simulink model "spike_generator"  (R2020b)
settings: Solver=FixedStepDiscrete  StartTime=0.0  StopTime=stopTime  RelTol=1e-3
InitFcn:
  | initCallback
StopFcn:
  | stopCallback
values from neighbouring files (symbols this model uses):
  nSites = 4    [Spike_Generator_Test_Parameters.m]
  tabs = 0.6e-3    (= 0.0006)    [Spike_Generator_Test_Parameters.m]
  trel = 0.6e-3    (= 0.0006)    [Spike_Generator_Test_Parameters.m]
undefined symbols (not defined in the file or in its folder): mp
settings Model: Creator=Ross  LastModifiedBy=tyler
settings DataIOCC: ReturnWorkspaceOutputs=off
settings OptimizationCC: BlockReduction=off  ConditionallyExecuteInputs=off  DefaultParameterBehavior=Inlined
settings DebuggingCC: ReadBeforeWriteMsg=DisableAll  WriteAfterWriteMsg=DisableAll  WriteAfterReadMsg=DisableAll  AlgebraicLoopMsg=error  MultiTaskDSMMsg=none  SingleTaskRateTransMsg=error  PregeneratedLibrarySubsystemCodeDiagnostic=none  ArithmeticOperatorsInVariantConditions=warning
settings HardwareCC: ProdBitPerPointer=32  ProdBitPerSizeT=32  ProdBitPerPtrDiffT=32  ProdLargestAtomicFloat=None  ProdIntDivRoundTo=Undefined  ProdEndianess=Unspecified  ProdWordSize=32  ProdHWDeviceType=ASIC/FPGA->ASIC/FPGA  TargetBitPerPointer=64  TargetBitPerSizeT=64  TargetBitPerPtrDiffT=64  TargetLongLongMode=on  TargetIntDivRoundTo=Zero  TargetEndianess=LittleEndian  TargetWordSize=64  TargetHWDeviceType=Custom Processor->MATLAB Host Computer  ProdEqTarget=off
settings ModelReferenceCC: UpdateModelReferenceTargets=IfOutOfDate
settings SFSimCC: SFSimEcho=off  SimUseLocalCustomCode=off  CustomCodeUndefinedFunction=UseInterfaceOnly
settings RTWCC: RTWUseLocalCustomCode=off

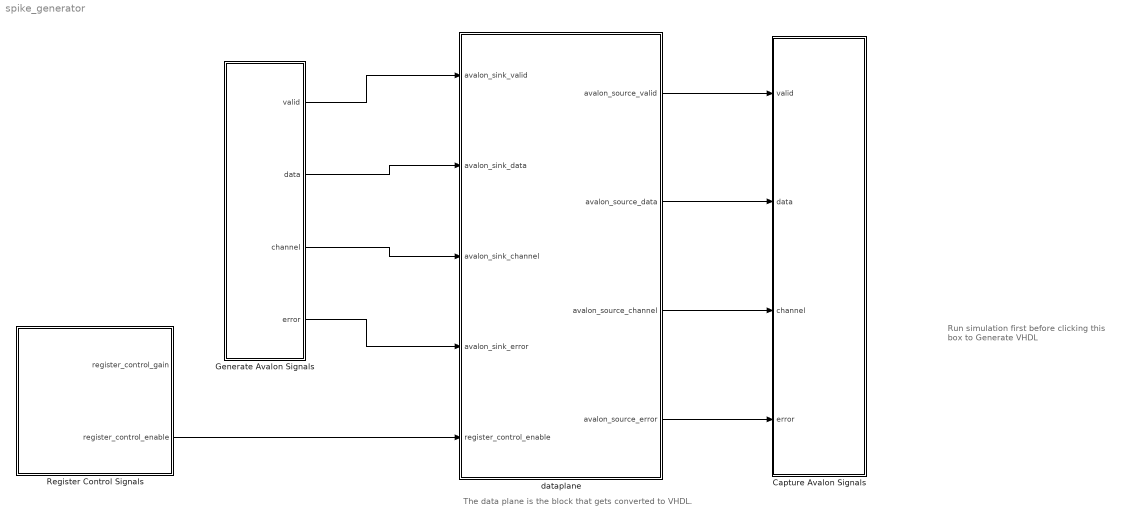
== system spike_generator ==
  note: The data plane is the block that gets converted to VHDL.
  note: Run simulation first
      | before clicking this box to
      | Generate VHDL
  Capture Avalon Signals : Subsystem
  Generate Avalon Signals : Subsystem
  Register Control Signals : Subsystem
  dataplane : Subsystem  TreatAsAtomicUnit=on
  wires:
  Generate Avalon Signals/2(data) -> dataplane/2(avalon_sink_data)
  Generate Avalon Signals/1(valid) -> dataplane/1(avalon_sink_valid)
  Generate Avalon Signals/3(channel) -> dataplane/3(avalon_sink_channel)
  Generate Avalon Signals/4(error) -> dataplane/4(avalon_sink_error)
  dataplane/2(avalon_source_data) -> Capture Avalon Signals/2(data)
  dataplane/1(avalon_source_valid) -> Capture Avalon Signals/1(valid)
  dataplane/3(avalon_source_channel) -> Capture Avalon Signals/3(channel)
  dataplane/4(avalon_source_error) -> Capture Avalon Signals/4(error)
  Register Control Signals/2(register_control_enable) -> dataplane/5(register_control_enable)

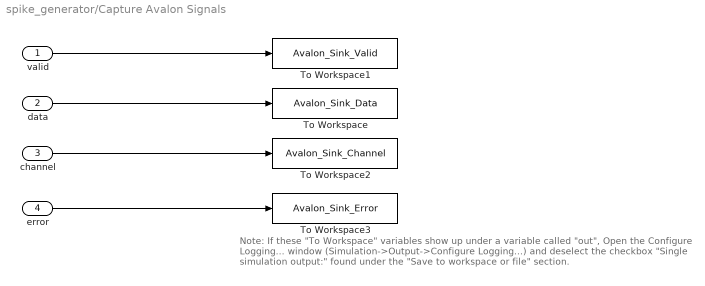
== system spike_generator/Capture Avalon Signals ==
  note: Note:  If these "To Workspace" variables show up under a variable called "out",
      | Open the Configure Logging... window (Simulation->Output->Configure Logging...)
      | and deselect the checkbox "Single simulation output:" found under the "Save to workspace or file" section.
  valid : Inport
  data : Inport  Port=2
  channel : Inport  Port=3
  error : Inport  Port=4
  To Workspace : ToWorkspace  VariableName=Avalon_Sink_Data  SaveFormat=Timeseries  SampleTime=-1
  To Workspace1 : ToWorkspace  VariableName=Avalon_Sink_Valid  SaveFormat=Timeseries  SampleTime=-1
  To Workspace2 : ToWorkspace  VariableName=Avalon_Sink_Channel  SaveFormat=Timeseries  SampleTime=-1
  To Workspace3 : ToWorkspace  VariableName=Avalon_Sink_Error  SaveFormat=Timeseries  SampleTime=-1
  wires:
  data/1 -> To Workspace/1
  valid/1 -> To Workspace1/1
  error/1 -> To Workspace3/1
  channel/1 -> To Workspace2/1

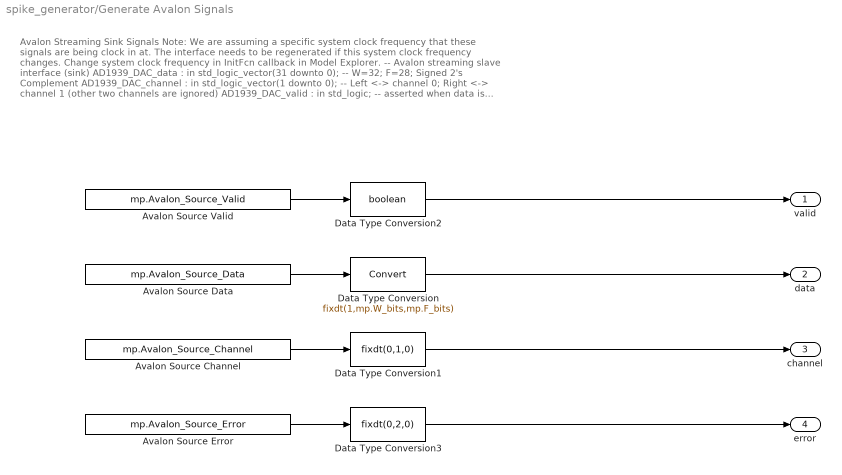
== system spike_generator/Generate Avalon Signals ==
  note: Avalon Streaming Sink Signals
      | Note: We are assuming a specific system clock frequency that these signals are being clock in at.
      | The interface needs to be regenerated if this system clock frequency changes. Change system clock frequency in InitFcn callback in Model Explorer.
      |
      | -- Avalon streaming slave interface (sink)
      | AD1939_DAC_data : in std_logic_vector(31 downto 0); -- W=32; F=28; Signed 2's Complement
      | AD1939_DAC_channel : in std_logic_vector(1 downto 0); -- Left <-> channel 0; Right <-> channel 1 (other two channels are ignored)
      | AD1939_DAC_valid : in std_logic; -- asserted when data is valid
      | AD1939_DAC_error : in std_logic_vector(1 downto 0) -- error channel is ignored, assumed to be error free at this point
      |
      | For more information on the data-channel-valid protocol, s ee chapter 5 in Intel's Avalon Interfaced Specification (p. 40) at https://www.intel.com/content/dam/www/programmable/us/en/pdfs/literature/manual/mnl_avalon_spec.pdf
  Avalon Source Channel : FromWorkspace  VariableName=mp.Avalon_Source_Channel  OutDataTypeStr=double  SampleTime=mp.Ts_sim
  "Avalon Source Data " : FromWorkspace  VariableName=mp.Avalon_Source_Data  OutDataTypeStr=double  SampleTime=mp.Ts_sim
  Avalon Source Error : FromWorkspace  VariableName=mp.Avalon_Source_Error  OutDataTypeStr=double  SampleTime=mp.Ts_sim
  Avalon Source Valid : FromWorkspace  VariableName=mp.Avalon_Source_Valid  OutDataTypeStr=double  SampleTime=mp.Ts_sim
  Data Type Conversion : DataTypeConversion  OutDataTypeStr=fixdt(1,mp.W_bits,mp.F_bits)
  Data Type Conversion1 : DataTypeConversion  OutDataTypeStr=fixdt(0,1,0)
  Data Type Conversion2 : DataTypeConversion  OutDataTypeStr=boolean
  Data Type Conversion3 : DataTypeConversion  OutDataTypeStr=fixdt(0,2,0)
  valid : Outport  VectorParamsAs1DForOutWhenUnconnected=off
  data : Outport  Port=2  VectorParamsAs1DForOutWhenUnconnected=off
  channel : Outport  Port=3  VectorParamsAs1DForOutWhenUnconnected=off
  error : Outport  Port=4  VectorParamsAs1DForOutWhenUnconnected=off
  wires:
  Data Type Conversion1/1 -> channel/1
  Data Type Conversion2/1 -> valid/1
  Avalon Source Error/1 -> Data Type Conversion3/1
  Data Type Conversion/1 -> data/1
  Avalon Source Valid/1 -> Data Type Conversion2/1
  Data Type Conversion3/1 -> error/1
  Avalon Source Channel/1 -> Data Type Conversion1/1
  "Avalon Source Data "/1 -> Data Type Conversion/1

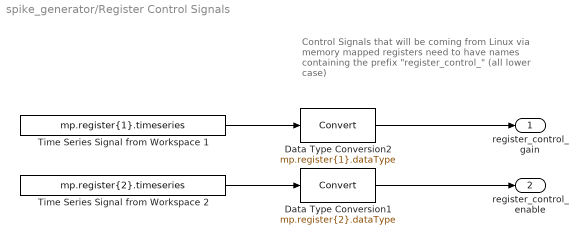
== system spike_generator/Register Control Signals ==
  note: Control Signals that will be coming from Linux via
      | memory mapped registers need to have names
      | containing the prefix "register_control_"
      | (all lower case)
  Data Type Conversion1 : DataTypeConversion  OutDataTypeStr=mp.register{2}.dataType
  Data Type Conversion2 : DataTypeConversion  OutDataTypeStr=mp.register{1}.dataType
  Time Series Signal from Workspace 1 : FromWorkspace  VariableName=mp.register{1}.timeseries  OutDataTypeStr=double  SampleTime=mp.Ts_sim
  Time Series Signal from Workspace 2 : FromWorkspace  VariableName=mp.register{2}.timeseries  OutDataTypeStr=double  SampleTime=mp.Ts_sim
  register_control_gain : Outport  VectorParamsAs1DForOutWhenUnconnected=off
  register_control_enable : Outport  Port=2  VectorParamsAs1DForOutWhenUnconnected=off
  wires:
  Time Series Signal from Workspace 1/1 -> Data Type Conversion2/1
  Data Type Conversion2/1 -> register_control_gain/1
  Data Type Conversion1/1 -> register_control_enable/1
  Time Series Signal from Workspace 2/1 -> Data Type Conversion1/1

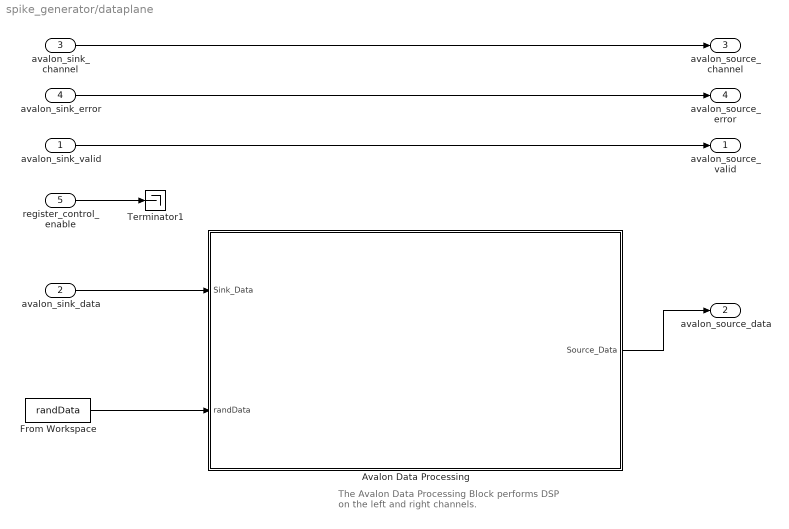
== system spike_generator/dataplane ==
  note: The Avalon Data Processing Block
      | performs DSP on the left and right channels.
  avalon_sink_valid : Inport
  avalon_sink_data : Inport  Port=2
  avalon_sink_channel : Inport  Port=3
  avalon_sink_error : Inport  Port=4
  register_control_enable : Inport  Port=5
  Avalon Data Processing : Subsystem  TreatAsAtomicUnit=on
  From Workspace : FromWorkspace  VariableName=randData
  Terminator1 : Terminator
  avalon_source_valid : Outport  VectorParamsAs1DForOutWhenUnconnected=off
  avalon_source_data : Outport  Port=2  VectorParamsAs1DForOutWhenUnconnected=off
  avalon_source_channel : Outport  Port=3  VectorParamsAs1DForOutWhenUnconnected=off
  avalon_source_error : Outport  Port=4  VectorParamsAs1DForOutWhenUnconnected=off
  wires:
  avalon_sink_error/1 -> avalon_source_error/1
  avalon_sink_valid/1 -> avalon_source_valid/1
  avalon_sink_data/1 -> Avalon Data Processing/1(Sink_Data)
  Avalon Data Processing/1(Source_Data) -> avalon_source_data/1
  avalon_sink_channel/1 -> avalon_source_channel/1
  register_control_enable/1 -> Terminator1/1
  From Workspace/1 -> Avalon Data Processing/2(randData)

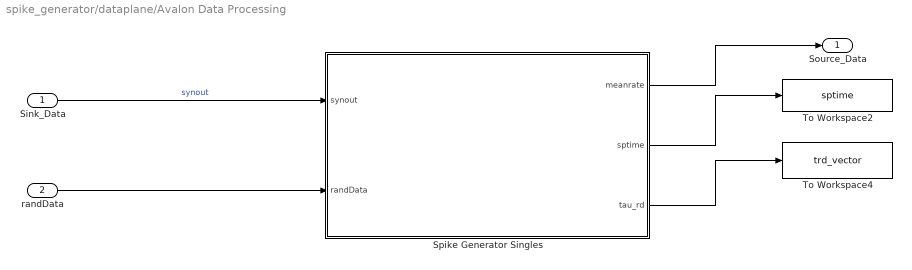
== system spike_generator/dataplane/Avalon Data Processing ==
  Sink_Data : Inport
  randData : Inport  Port=2
  Spike Generator Singles : Subsystem
  To Workspace2 : ToWorkspace  VariableName=sptime  SampleTime=-1
      settings: Save2DSignal=2-D array (concatenate along first dimension)
  To Workspace4 : ToWorkspace  VariableName=trd_vector  SampleTime=-1
      settings: Save2DSignal=2-D array (concatenate along first dimension)
  Source_Data : Outport  InitialOutput=0  VectorParamsAs1DForOutWhenUnconnected=off
  wires:
  Sink_Data/1 -> Spike Generator Singles/1(synout)  "synout"
  Spike Generator Singles/1(meanrate) -> Source_Data/1
  Spike Generator Singles/3(tau_rd) -> To Workspace4/1
  randData/1 -> Spike Generator Singles/2(randData)
  Spike Generator Singles/2(sptime) -> To Workspace2/1

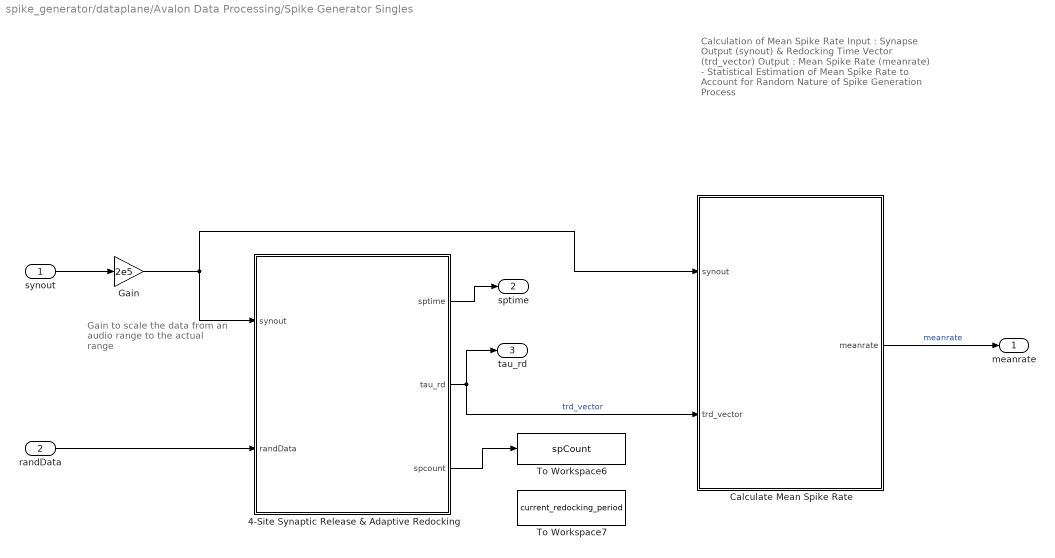
== system spike_generator/dataplane/Avalon Data Processing/Spike Generator Singles ==
  note: Gain to scale the
      | data from an audio
      | range to the actual
      | range
  note: Calculation of Mean Spike Rate
      |
      | Input : Synapse Output (synout) & Redocking Time Vector (trd_vector)
      |
      | Output : Mean Spike Rate (meanrate)
      |
      | - Statistical Estimation of Mean Spike Rate to Account for Random Nature of Spike Generation Process
  synout : Inport
  randData : Inport  Port=2
  4-Site Synaptic Release & Adaptive Redocking : Subsystem
  Calculate Mean Spike Rate : Subsystem
  Gain : Gain  Gain=2e5
  To Workspace6 : ToWorkspace  VariableName=spCount  SampleTime=-1
      settings: Save2DSignal=2-D array (concatenate along first dimension)
  To Workspace7 : ToWorkspace  VariableName=current_redocking_period  SampleTime=-1
      settings: Save2DSignal=2-D array (concatenate along first dimension)
  meanrate : Outport
  sptime : Outport  Port=2
  tau_rd : Outport  Port=3
  wires:
  4-Site Synaptic Release & Adaptive Redocking/2(tau_rd) -> tau_rd/1, Calculate Mean Spike Rate/2(trd_vector)  "trd_vector"
  Calculate Mean Spike Rate/1(meanrate) -> meanrate/1  "meanrate"
  randData/1 -> 4-Site Synaptic Release & Adaptive Redocking/2(randData)
  4-Site Synaptic Release & Adaptive Redocking/1(sptime) -> sptime/1
  synout/1 -> Gain/1
  Gain/1 -> Calculate Mean Spike Rate/1(synout), 4-Site Synaptic Release & Adaptive Redocking/1(synout)
  4-Site Synaptic Release & Adaptive Redocking/3(spcount) -> To Workspace6/1
  ? -> To Workspace7/1

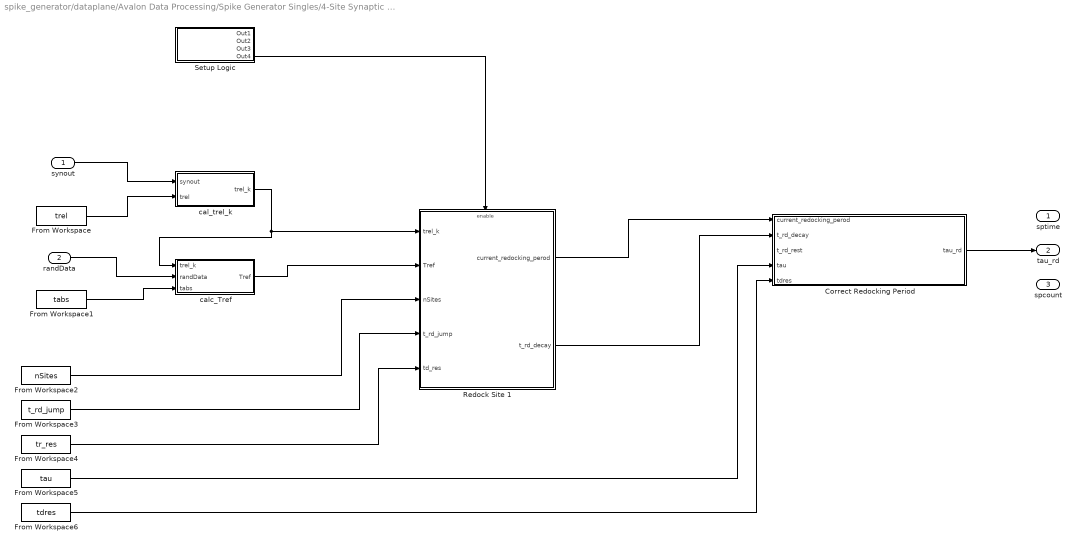
== system spike_generator/dataplane/Avalon Data Processing/Spike Generator Singles/4-Site Synaptic Release & Adaptive Redocking ==
  synout : Inport
  randData : Inport  Port=2
  Correct Redocking Period : Subsystem
  From Workspace : FromWorkspace  VariableName=trel  OutputAfterFinalValue=Holding final value
  From Workspace1 : FromWorkspace  VariableName=tabs  OutputAfterFinalValue=Holding final value
  From Workspace2 : FromWorkspace  VariableName=nSites  OutputAfterFinalValue=Holding final value
  From Workspace3 : FromWorkspace  VariableName=t_rd_jump  OutputAfterFinalValue=Holding final value
  From Workspace4 : FromWorkspace  VariableName=tr_res  OutputAfterFinalValue=Holding final value
  From Workspace5 : FromWorkspace  VariableName=tau
  From Workspace6 : FromWorkspace  VariableName=tdres
  Redock Site 1 : Subsystem  TreatAsAtomicUnit=on
  Setup Logic : Subsystem
  cal_trel_k : Subsystem
  calc_Tref : Subsystem
  sptime : Outport
  tau_rd : Outport  Port=2
  spcount : Outport  Port=3
  wires:
  From Workspace/1 -> cal_trel_k/2(trel)
  synout/1 -> cal_trel_k/1(synout)
  cal_trel_k/1(trel_k) -> calc_Tref/1(trel_k), Redock Site 1/1(trel_k)
  From Workspace1/1 -> calc_Tref/3(tabs)
  randData/1 -> calc_Tref/2(randData)
  From Workspace2/1 -> Redock Site 1/3(nSites)
  calc_Tref/1(Tref) -> Redock Site 1/2(Tref)
  Setup Logic/4(Out4) -> Redock Site 1/Enable
  From Workspace3/1 -> Redock Site 1/4(t_rd_jump)
  From Workspace4/1 -> Redock Site 1/5(td_res)
  Redock Site 1/1(current_redocking_perod) -> Correct Redocking Period/1(current_redocking_perod)
  Correct Redocking Period/1(tau_rd) -> tau_rd/1
  Redock Site 1/2(t_rd_decay) -> Correct Redocking Period/2(t_rd_decay)
  From Workspace5/1 -> Correct Redocking Period/4(tau)
  From Workspace6/1 -> Correct Redocking Period/5(tdres)

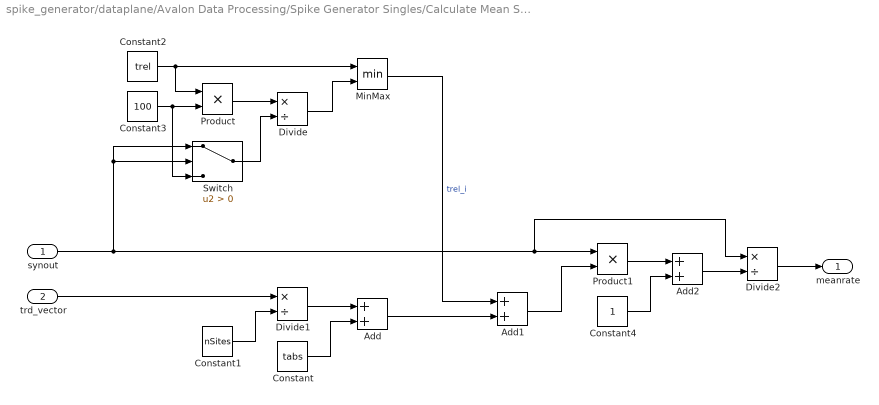
== system spike_generator/dataplane/Avalon Data Processing/Spike Generator Singles/Calculate Mean Spike Rate ==
  synout : Inport
  trd_vector : Inport  Port=2
  Add : Sum
  Add1 : Sum
  Add2 : Sum
  Constant : Constant  Value=tabs  OutDataTypeStr=single  SampleTime=-1
  Constant1 : Constant  Value=nSites  OutDataTypeStr=single  SampleTime=-1
  Constant2 : Constant  Value=trel  OutDataTypeStr=single  SampleTime=-1
  Constant3 : Constant  Value=100  OutDataTypeStr=single  SampleTime=-1
  Constant4 : Constant  OutDataTypeStr=single  SampleTime=-1
  Divide : Product  Inputs=*/  RndMeth=Zero  SaturateOnIntegerOverflow=on
  Divide1 : Product  Inputs=*/  RndMeth=Zero  SaturateOnIntegerOverflow=on
  Divide2 : Product  Inputs=*/  RndMeth=Zero  SaturateOnIntegerOverflow=on
  MinMax : MinMax  Inputs=2
  Product : Product
  Product1 : Product
  Switch : Switch  Criteria=u2 > Threshold
  meanrate : Outport  VectorParamsAs1DForOutWhenUnconnected=off
  wires:
  synout/1 -> Switch/1, Switch/2, Divide2/1, Product1/1
  trd_vector/1 -> Divide1/1
  Constant2/1 -> MinMax/1, Product/1
  Constant3/1 -> Switch/3, Product/2
  Product/1 -> Divide/1
  Divide/1 -> MinMax/2
  MinMax/1 -> Add1/1  "trel_i"
  Constant1/1 -> Divide1/2
  Divide1/1 -> Add/1
  Constant/1 -> Add/2
  Add/1 -> Add1/2
  Constant4/1 -> Add2/2
  Add1/1 -> Product1/2
  Product1/1 -> Add2/1
  Add2/1 -> Divide2/2
  Divide2/1 -> meanrate/1
  Switch/1 -> Divide/2

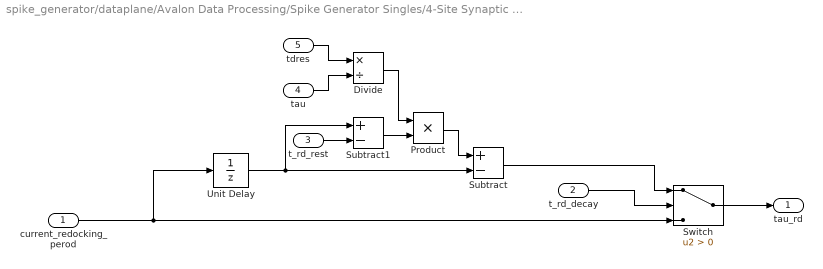
== system spike_generator/dataplane/Avalon Data Processing/Spike Generator Singles/4-Site Synaptic Release & Adaptive Redocking/Correct Redocking Period ==
  current_redocking_perod : Inport
  t_rd_decay : Inport  Port=2
  t_rd_rest : Inport  Port=3
  tau : Inport  Port=4
  tdres : Inport  Port=5
  Divide : Product  Inputs=*/
  Product : Product
  Subtract : Sum  Inputs=+-
  Subtract1 : Sum  Inputs=+-
  Switch : Switch  Criteria=u2 > Threshold
  Unit Delay : UnitDelay  SampleTime=-1  HasFrameUpgradeWarning=on
  tau_rd : Outport
  wires:
  current_redocking_perod/1 -> Switch/3, Unit Delay/1
  t_rd_decay/1 -> Switch/2
  Switch/1 -> tau_rd/1
  Unit Delay/1 -> Subtract1/1, Subtract/2
  tdres/1 -> Divide/1
  tau/1 -> Divide/2
  t_rd_rest/1 -> Subtract1/2
  Divide/1 -> Product/1
  Subtract1/1 -> Product/2
  Product/1 -> Subtract/1
  Subtract/1 -> Switch/1

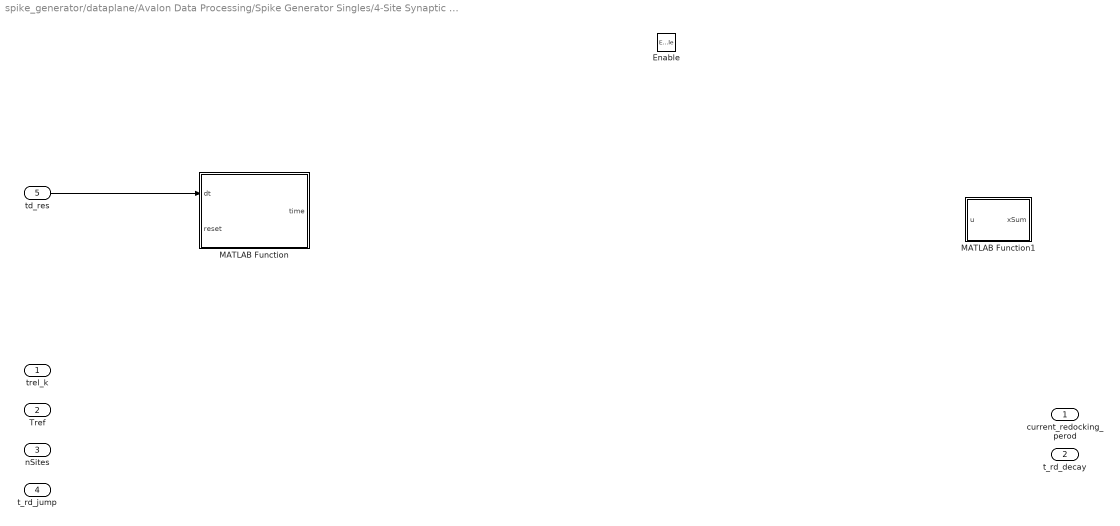
== system spike_generator/dataplane/Avalon Data Processing/Spike Generator Singles/4-Site Synaptic Release & Adaptive Redocking/Redock Site 1 ==
  trel_k : Inport
  Tref : Inport  Port=2
  nSites : Inport  Port=3
  t_rd_jump : Inport  Port=4
  td_res : Inport  Port=5
  Enable : EnablePort
  MATLAB Function : MATLAB Function  TreatAsAtomicUnit=on
  MATLAB Function1 : MATLAB Function  TreatAsAtomicUnit=on
  current_redocking_perod : Outport
  t_rd_decay : Outport  Port=2
  wires:
  td_res/1 -> MATLAB Function/1(dt)

== system spike_generator/dataplane/Avalon Data Processing/Spike Generator Singles/4-Site Synaptic Release & Adaptive Redocking/Setup Logic ==
  Constant : Constant  OutDataTypeStr=boolean  SampleTime=-1
  Out1 : Outport
  Out2 : Outport  Port=2
  Out3 : Outport  Port=3
  Out4 : Outport  Port=4
  wires:
  Constant/1 -> Out1/1, Out2/1, Out3/1, Out4/1

== system spike_generator/dataplane/Avalon Data Processing/Spike Generator Singles/4-Site Synaptic Release & Adaptive Redocking/cal_trel_k ==
  synout : Inport
  trel : Inport  Port=2
  Divide : Product  Inputs=*/
  K : Gain  Gain=100
  Min : MinMax  Inputs=2
  trel_k : Outport
  wires:
  Divide/1 -> Min/1
  Min/1 -> trel_k/1
  K/1 -> Divide/1
  trel/1 -> K/1, Min/2
  synout/1 -> Divide/2

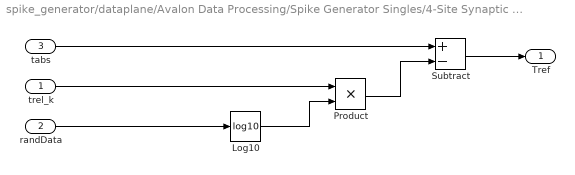
== system spike_generator/dataplane/Avalon Data Processing/Spike Generator Singles/4-Site Synaptic Release & Adaptive Redocking/calc_Tref ==
  trel_k : Inport
  randData : Inport  Port=2
  tabs : Inport  Port=3
  Log10 : Math  Operator=log10  SaturateOnIntegerOverflow=on
  Product : Product
  Subtract : Sum  Inputs=+-
  Tref : Outport
  wires:
  tabs/1 -> Subtract/1
  randData/1 -> Log10/1
  trel_k/1 -> Product/1
  Log10/1 -> Product/2
  Product/1 -> Subtract/2
  Subtract/1 -> Tref/1

== matlab function spike_generator/dataplane/Avalon Data Processing/Spike Generator Singles/4-Site Synaptic Release & Adaptive Redocking/Redock Site 1/MATLAB Function ==
  data: time output; dt input; reset input
function time = increment_time(dt,reset)
  persistent elapsed_time
  
  if isempty(elapsed_time)
    elapsed_time = 0;
  end
  if reset == 0
    elapsed_time = elapsed_time + dt;
  else
    elapsed_time = 0;
  end
  time = elapsed_time;
end

== matlab function spike_generator/dataplane/Avalon Data Processing/Spike Generator Singles/4-Site Synaptic Release & Adaptive Redocking/Redock Site 1/MATLAB Function1 ==
  data: u input; xSum output
function xSum = fcn(u)

y = u;
